simulink model "STATE_PROJECT_Harness_Test_4"  (R2022b)
settings: Solver=FixedStepAuto  StartTime=0.0  StopTime=120.0  FixedStep=0.1  RelTol=1e-3
settings Model: NumberOfSteps=10  Creator=giuse  LastModifiedBy=giuse

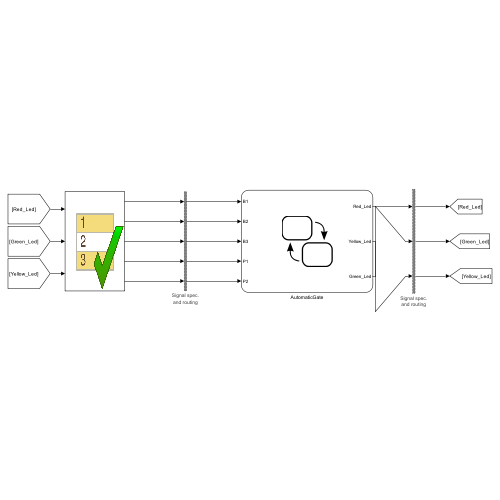
[thumbnail: Simulink's stored preview of the top-level diagram]
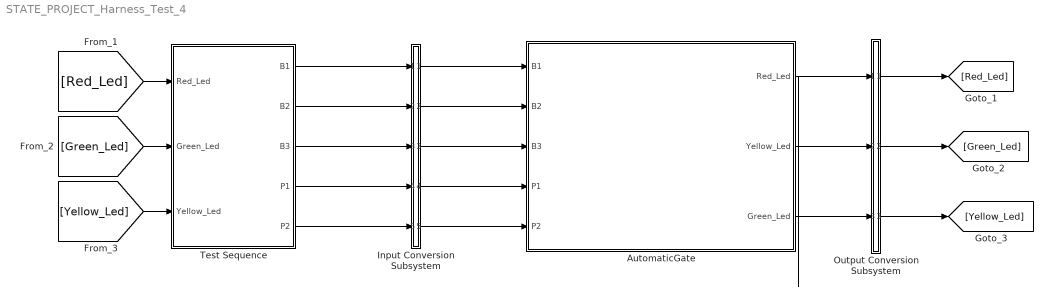
== system STATE_PROJECT_Harness_Test_4 ==
  AutomaticGate : Stateflow chart  TreatAsAtomicUnit=on
      settings: PortSchema="{\"entries\":[{\"content\":{\"sides\":[{\"content\":{\"connectorIds\":[\"In1\",\"In2\",\"In3\",\"In4\",\"In5\"]},\"type\":\"ConnectorPlacement.EquallySpacedRectSide\",\"uuid\":\"b9ac80a2-bb7a-47d7-8c7f-6386963f3ff2\"},{\"content\":{\"connectorIds\":[\"Out1\",\"Out3\",\"Out2\"],\"side\":\"RIGHT\"},\"type\":\"ConnectorPlacement.EquallySpacedRectSide\",\"uuid\":\"565990b0-d594-46a7-8ea3-0c7443a62f81\"},{\"content\":{\"connectorIds\":[],\"side\":\"TOP\"},\"type\":\"ConnectorPlacement.EquallySpacedRectSide\",\"uuid\":\"d7a99aca-bf8f-44a8-855e-79befe08fc9b\"}]},\"type\":\"ConnectorPlacement.EquallySpacedConnector\",\"uuid\":\"af0d90d0-169d-45ca-9585-d3b64258f7d0\"}],\"packageUris\":[\"http://schema.mathworks.com/mf0/Connector/R2020b\"],\"version\":\"1.0\"}"
  Input Conversion Subsystem : Subsystem  Tag=__SLT_ICS__  Description=|
      | Signal spec.
      | and routing
      settings: AttributesFormatString=%<Description>
  Output Conversion Subsystem : Subsystem  Tag=__SLT_OCS__  Description=|
      | Signal spec.
      | and routing
      settings: AttributesFormatString=%<Description>
  Test Sequence : Test Sequence  TreatAsAtomicUnit=on
  wires:
  Test Sequence/1(B1) -> Input Conversion Subsystem/1(Inport_1)
  Test Sequence/2(B2) -> Input Conversion Subsystem/2(Inport_2)
  Test Sequence/3(B3) -> Input Conversion Subsystem/3(Inport_3)
  Test Sequence/4(P1) -> Input Conversion Subsystem/4(Inport_4)
  Test Sequence/5(P2) -> Input Conversion Subsystem/5(Inport_5)
  [Red_Led] -> Test Sequence/1(Red_Led)
  [Green_Led] -> Test Sequence/2(Green_Led)
  [Yellow_Led] -> Test Sequence/3(Yellow_Led)
  Output Conversion Subsystem/1(Outport_1) -> [Red_Led]
  Output Conversion Subsystem/2(Outport_2) -> [Green_Led]
  Output Conversion Subsystem/3(Outport_3) -> [Yellow_Led]
  Input Conversion Subsystem/1(Outport_1) -> AutomaticGate/1(B1)
  Input Conversion Subsystem/2(Outport_2) -> AutomaticGate/2(B2)
  Input Conversion Subsystem/3(Outport_3) -> AutomaticGate/3(B3)
  Input Conversion Subsystem/4(Outport_4) -> AutomaticGate/4(P1)
  Input Conversion Subsystem/5(Outport_5) -> AutomaticGate/5(P2)
  AutomaticGate/1(Red_Led) -> Output Conversion Subsystem/1(Inport_1)
  AutomaticGate/2(Green_Led) -> Output Conversion Subsystem/2(Inport_2)
  AutomaticGate/3(Yellow_Led) -> Output Conversion Subsystem/3(Inport_3)

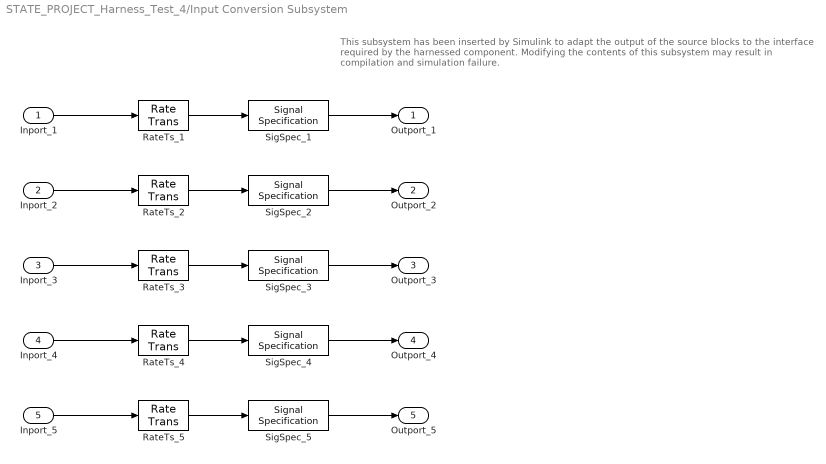
== system STATE_PROJECT_Harness_Test_4/Input Conversion Subsystem ==
  note: This subsystem has been inserted by Simulink to adapt the output of the source blocks to the interface required by the harnessed component.
      |  Modifying the contents of this subsystem may result in compilation and simulation failure.
  Inport_1 : Inport
  Inport_2 : Inport  Port=2
  Inport_3 : Inport  Port=3
  Inport_4 : Inport  Port=4
  Inport_5 : Inport  Port=5
  RateTs_{1..3,5} (4 alike) : RateTransition  OutPortSampleTime=0.1
  RateTs_4 : RateTransition  OutPortSampleTime=[-1, 0]
  SigSpec_{1..3,5} (4 alike) : SignalSpecification  OutDataTypeStr=double  Dimensions=[1]  SampleTime=0.1
  SigSpec_4 : SignalSpecification  OutDataTypeStr=double  Dimensions=[1]  SampleTime=[-1, 0]
  Outport_1 : Outport
  Outport_2 : Outport  Port=2
  Outport_3 : Outport  Port=3
  Outport_4 : Outport  Port=4
  Outport_5 : Outport  Port=5
  wires:
  SigSpec_1/1 -> Outport_1/1
  RateTs_1/1 -> SigSpec_1/1
  Inport_1/1 -> RateTs_1/1
  SigSpec_2/1 -> Outport_2/1
  RateTs_2/1 -> SigSpec_2/1
  Inport_2/1 -> RateTs_2/1
  SigSpec_3/1 -> Outport_3/1
  RateTs_3/1 -> SigSpec_3/1
  Inport_3/1 -> RateTs_3/1
  SigSpec_4/1 -> Outport_4/1
  RateTs_4/1 -> SigSpec_4/1
  Inport_4/1 -> RateTs_4/1
  SigSpec_5/1 -> Outport_5/1
  RateTs_5/1 -> SigSpec_5/1
  Inport_5/1 -> RateTs_5/1

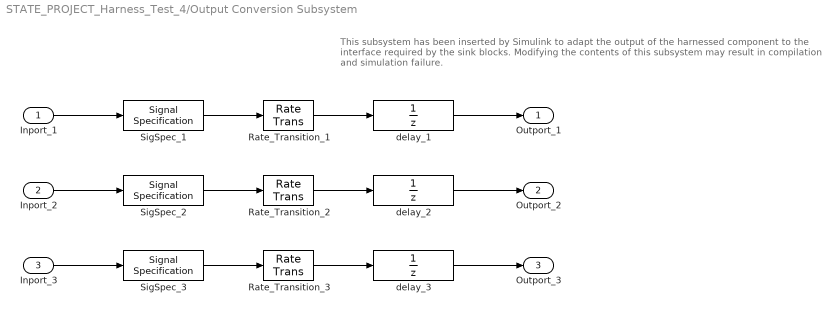
== system STATE_PROJECT_Harness_Test_4/Output Conversion Subsystem ==
  note: This subsystem has been inserted by Simulink to adapt the output of the harnessed component to the interface required by the sink blocks.
      |  Modifying the contents of this subsystem may result in compilation and simulation failure.
  Inport_1 : Inport
  Inport_2 : Inport  Port=2
  Inport_3 : Inport  Port=3
  Rate_Transition_1 : RateTransition  OutPortSampleTimeOpt=Inherit
  Rate_Transition_2 : RateTransition  OutPortSampleTimeOpt=Inherit
  Rate_Transition_3 : RateTransition  OutPortSampleTimeOpt=Inherit
  SigSpec_1 : SignalSpecification  OutDataTypeStr=double  Dimensions=[1]  SampleTime=0.1
  SigSpec_2 : SignalSpecification  OutDataTypeStr=double  Dimensions=[1]  SampleTime=0.1
  SigSpec_3 : SignalSpecification  OutDataTypeStr=double  Dimensions=[1]  SampleTime=0.1
  delay_1 : UnitDelay  SampleTime=-1
  delay_2 : UnitDelay  SampleTime=-1
  delay_3 : UnitDelay  SampleTime=-1
  Outport_1 : Outport
  Outport_2 : Outport  Port=2
  Outport_3 : Outport  Port=3
  wires:
  Inport_1/1 -> SigSpec_1/1
  SigSpec_1/1 -> Rate_Transition_1/1
  Rate_Transition_1/1 -> delay_1/1
  delay_1/1 -> Outport_1/1
  Inport_2/1 -> SigSpec_2/1
  SigSpec_2/1 -> Rate_Transition_2/1
  Rate_Transition_2/1 -> delay_2/1
  delay_2/1 -> Outport_2/1
  Inport_3/1 -> SigSpec_3/1
  SigSpec_3/1 -> Rate_Transition_3/1
  Rate_Transition_3/1 -> delay_3/1
  delay_3/1 -> Outport_3/1

== stateflow chart STATE_PROJECT_Harness_Test_4/AutomaticGate ==
  state AUTOMATIC_GATE_LOGIC
    state AUTOMATIC_GATE [parallel]
      settings: executionOrder=4
      state EMERGENCY_P1_CLOSED
        state GREEN_OFF
          en:
          Green_Led = LED_OFF;
          Yellow_Led = LED_OFF;
          Red_Led = LED_OFF;
        state GREEN_ON
          en:
          Green_Led = LED_ON;
          Yellow_Led = LED_OFF;
          Red_Led = LED_OFF;
        AUTOMATIC_GATE_LOGIC.AUTOMATIC_GATE.EMERGENCY_P1_CLOSED.GREEN_ON -> AUTOMATIC_GATE_LOGIC.AUTOMATIC_GATE.EMERGENCY_P1_CLOSED.GREEN_OFF : [after(GREEN_DUR,sec)]
        AUTOMATIC_GATE_LOGIC.AUTOMATIC_GATE.EMERGENCY_P1_CLOSED.GREEN_OFF -> AUTOMATIC_GATE_LOGIC.AUTOMATIC_GATE.EMERGENCY_P1_CLOSED.GREEN_ON : [after(GREEN_DUR,sec)]
        (default) -> AUTOMATIC_GATE_LOGIC.AUTOMATIC_GATE.EMERGENCY_P1_CLOSED.GREEN_ON
      state CLOSED
        en:
        Green_Led = LED_OFF;
        Yellow_Led = LED_OFF;
        Red_Led = LED_OFF;
        state WORK_DUR_SETTING [parallel]
          settings: executionOrder=2
          state WORK_DUR_SETTING_INTERNAL
          (default) -> WORK_DUR_SETTING_INTERNAL
          WORK_DUR_SETTING_INTERNAL -> WORK_DUR_SETTING_INTERNAL : B3_pressed{WORK_DUR = mod((WORK_DUR),120) +10;}
        state OPEN_DUR_SETTING [parallel]
          settings: executionOrder=1
          state OPEN_DUR_SETTING_INTERNAL
          OPEN_DUR_SETTING_INTERNAL -> OPEN_DUR_SETTING_INTERNAL : B2_pressed{OPEN_DUR = mod((OPEN_DUR),120) + 10;}
        (default) -> WORK_DUR_SETTING [order 2]
        (default) -> OPEN_DUR_SETTING [order 1]
      state OPENING
        state YELLOW_OFF
          en:
          Green_Led = LED_OFF;
          Yellow_Led = LED_OFF;
          Red_Led = LED_OFF;
        state YELLOW_ON
          en:
          Green_Led = LED_OFF;
          Yellow_Led = LED_ON;
          Red_Led = LED_OFF;
        AUTOMATIC_GATE_LOGIC.AUTOMATIC_GATE.OPENING.YELLOW_ON -> AUTOMATIC_GATE_LOGIC.AUTOMATIC_GATE.OPENING.YELLOW_OFF : [after(YELLOW_DUR,sec)]
        AUTOMATIC_GATE_LOGIC.AUTOMATIC_GATE.OPENING.YELLOW_OFF -> AUTOMATIC_GATE_LOGIC.AUTOMATIC_GATE.OPENING.YELLOW_ON : [after(YELLOW_DUR,sec)]
        (default) -> AUTOMATIC_GATE_LOGIC.AUTOMATIC_GATE.OPENING.YELLOW_ON
      state EMERGENCY
        en:
        Green_Led = LED_OFF;
        Yellow_Led = LED_OFF;
        Red_Led = LED_OFF;
      state EMERGENCY_LED
        en:
        Green_Led = LED_OFF;
        Yellow_Led = LED_OFF;
        Red_Led = LED_ON;
      state CLOSING
        state YELLOW_OFF
          en:
          Green_Led = LED_OFF;
          Yellow_Led = LED_OFF;
          Red_Led = LED_OFF;
        state YELLOW_ON
          en:
          Green_Led = LED_OFF;
          Yellow_Led = LED_ON;
          Red_Led = LED_OFF;
        AUTOMATIC_GATE_LOGIC.AUTOMATIC_GATE.CLOSING.YELLOW_ON -> AUTOMATIC_GATE_LOGIC.AUTOMATIC_GATE.CLOSING.YELLOW_OFF : [after(YELLOW_DUR,sec)]
        AUTOMATIC_GATE_LOGIC.AUTOMATIC_GATE.CLOSING.YELLOW_OFF -> AUTOMATIC_GATE_LOGIC.AUTOMATIC_GATE.CLOSING.YELLOW_ON : [after(YELLOW_DUR,sec)]
        (default) -> AUTOMATIC_GATE_LOGIC.AUTOMATIC_GATE.CLOSING.YELLOW_ON
      state OPEN
        en:
        Green_Led = LED_ON;
        Yellow_Led = LED_ON;
        Red_Led = LED_ON;
      state EMERGENCY_P1_OPEN
        state GREEN_OFF
          en:
          Green_Led = LED_OFF;
          Yellow_Led = LED_OFF;
          Red_Led = LED_OFF;
        state GREEN_ON
          en:
          Green_Led = LED_ON;
          Yellow_Led = LED_OFF;
          Red_Led = LED_OFF;
        AUTOMATIC_GATE_LOGIC.AUTOMATIC_GATE.EMERGENCY_P1_OPEN.GREEN_ON -> AUTOMATIC_GATE_LOGIC.AUTOMATIC_GATE.EMERGENCY_P1_OPEN.GREEN_OFF : [after(GREEN_DUR,sec)]
        AUTOMATIC_GATE_LOGIC.AUTOMATIC_GATE.EMERGENCY_P1_OPEN.GREEN_OFF -> AUTOMATIC_GATE_LOGIC.AUTOMATIC_GATE.EMERGENCY_P1_OPEN.GREEN_ON : [after(GREEN_DUR,sec)]
        (default) -> AUTOMATIC_GATE_LOGIC.AUTOMATIC_GATE.EMERGENCY_P1_OPEN.GREEN_ON
      CLOSED -> EMERGENCY_P1_CLOSED [order 1] : [B1_pressed && P1 == P_ON]
      EMERGENCY_P1_CLOSED -> CLOSED : [P1 == P_OFF || after(EMER_P1_DUR,sec)]
      CLOSED -> OPENING [order 2] : B1_pressed
      EMERGENCY -> CLOSED [order 2] : [P2 == P_ON]
      EMERGENCY_LED -> CLOSED : [P2 == P_ON]
      CLOSING -> CLOSED [order 1] : [P2 == P_ON]
      EMERGENCY -> EMERGENCY_LED [order 1] : [after(EMER_DUR,sec)]
      CLOSING -> EMERGENCY [order 3] : [after(WORK_DUR,sec)]
      OPENING -> CLOSING [order 1] : [B1_pressed && P1 == P_OFF]
      CLOSING -> OPENING [order 2] : [B1_pressed || P1 == P_ON]
      OPENING -> OPEN [order 2] : [after(WORK_DUR,sec)]
      (default) -> CLOSING
      OPEN -> CLOSING [order 1] : [after(OPEN_DUR,sec) || B1_pressed]
      EMERGENCY_P1_OPEN -> OPEN : [P1 == P_OFF || after(EMER_P1_DUR,sec)]
      OPEN -> EMERGENCY_P1_OPEN [order 2] : [B1_pressed && P1 == P_ON]
    state B1 [parallel]
      settings: executionOrder=1
      state RELEASED
      state PRESSED
      state LONGPRESSED
        send(B1_pressed)
      (default) -> AUTOMATIC_GATE_LOGIC.B1.RELEASED
      AUTOMATIC_GATE_LOGIC.B1.RELEASED -> AUTOMATIC_GATE_LOGIC.B1.PRESSED : [B1==BUTTON_ON]
      AUTOMATIC_GATE_LOGIC.B1.LONGPRESSED -> AUTOMATIC_GATE_LOGIC.B1.RELEASED : [B1 == BUTTON_OFF]
      AUTOMATIC_GATE_LOGIC.B1.PRESSED -> AUTOMATIC_GATE_LOGIC.B1.LONGPRESSED : [B1 == BUTTON_OFF]
    state B3 [parallel]
      settings: executionOrder=2
      state RELEASED
      state PRESSED
      state LONGPRESSED
        send(B3_pressed)
      (default) -> AUTOMATIC_GATE_LOGIC.B3.RELEASED
      AUTOMATIC_GATE_LOGIC.B3.RELEASED -> AUTOMATIC_GATE_LOGIC.B3.PRESSED : [B3==BUTTON_ON]
      AUTOMATIC_GATE_LOGIC.B3.LONGPRESSED -> AUTOMATIC_GATE_LOGIC.B3.RELEASED : [B3 == BUTTON_OFF]
      AUTOMATIC_GATE_LOGIC.B3.PRESSED -> AUTOMATIC_GATE_LOGIC.B3.LONGPRESSED : [B3== BUTTON_OFF]
    state B2 [parallel]
      settings: executionOrder=3
      state RELEASED
      state PRESSED
      state LONGPRESSED
        send(B2_pressed)
      (default) -> AUTOMATIC_GATE_LOGIC.B2.RELEASED
      AUTOMATIC_GATE_LOGIC.B2.RELEASED -> AUTOMATIC_GATE_LOGIC.B2.PRESSED : [B2==BUTTON_ON]
      AUTOMATIC_GATE_LOGIC.B2.LONGPRESSED -> AUTOMATIC_GATE_LOGIC.B2.RELEASED : [B2 == BUTTON_OFF]
      AUTOMATIC_GATE_LOGIC.B2.PRESSED -> AUTOMATIC_GATE_LOGIC.B2.LONGPRESSED : [B2 == BUTTON_OFF]
    (default) -> AUTOMATIC_GATE [order 1]
    (default) -> B1 [order 2]
    (default) -> B3 [order 4]
    (default) -> B2 [order 3]
  data: B1 input; B2 input; B3 input; Red_Led output; Green_Led output; Yellow_Led output; P1 input; P2 input; BUTTON_OFF constant double =0; WORK_DUR local =10; P_ON constant double =1; P_OFF constant double =0; OPEN_DUR local =10; LED_ON constant double =1; LED_OFF constant double =0; BUTTON_ON constant double =1; EMER_DUR constant double =10; YELLOW_DUR constant double =1; GREEN_DUR constant double =0.5; EMER_P1_DUR constant double =30
  events: B1_pressed local RISING_EDGE_EVENT; B2_pressed local FUNCTION_CALL_EVENT; B3_pressed local FUNCTION_CALL_EVENT

== stateflow chart STATE_PROJECT_Harness_Test_4/Test Sequence ==
  settings: updateMethod=DISCRETE  sampleTime=0.1
  state Run
    %% Initialize data outputs.
    B1 = 0;
    B2 = 0;
    B3 = 0;
    P1 = 0;
    P2 = 0;
    settings: description=Inizializzazione degli input
  state Test_closing_state
    settings: description=Test dello sato di chiusura intercendo gli stati del Led_Yellow
    state Test_closing_state_1
      verify(Yellow_Led == 1, 'TEST FAILED');
      settings: description=Yellow_Led == ON
    state Test_closing_state_2
      verify(Yellow_Led == 0, 'TEST FAILED');
      settings: description=Yellow_Led == OFF
    (default) -> Test_closing_state_1
    Test_closing_state_1 -> Test_closing_state_2 : [
        | after(1,sec)
        | ]
    Test_closing_state_2 -> Test_closing_state_1 : [
        | after(1,sec)
        | ]
  state Start_test_P1
    P1=1;
    settings: description=|
        | Inizializzazione variabile per andare nello stato di OPENING, a cusa dell'ostacolo
        | davanti a P1
  state Test_opening_state
    settings: description=Test dello sato di apertura intercendo gli stati del Led_Yellow
    state Start_test_opening_1
      verify(Yellow_Led == 1, 'TEST FAILED');
      settings: description=Yellow_Led == ON
    state Start_test_opening_2
      verify(Yellow_Led == 0, 'TEST FAILED');
      settings: description=Yellow_Led == OFF
    (default) -> Start_test_opening_1
    Start_test_opening_1 -> Start_test_opening_2 : [
        | after(1,sec)
        | ]
    Start_test_opening_2 -> Start_test_opening_1 : [
        | after(1,sec)
        | ]
  state Test_open_state
    verify(Green_Led == 1, 'TEST FAILED');
    verify(Yellow_Led == 1, 'TEST FAILED');
    verify(Red_Led == 1, 'TEST FAILED');
    settings: description=Testinf dello stato OPEN verificando che tutti i led sono accesi
  state Test_change_P1
    P1=0;
    settings: description=Inizializzazione sensore P1 a 0 per togliere l'ostacolo
  state Start_test_closing_state
    settings: description="Genera fronte di salita e discesa del pulsante B1 per cambiare da stato OPEN  A CLOSING"
    state Start_test_closing_state_1
      B1=1;
      settings: description=B1 = 1
    state Start_test_closing_state_2
      B1=0;
      settings: description=B1 = 0
    (default) -> Start_test_closing_state_1
    Start_test_closing_state_1 -> Start_test_closing_state_2 : [
        | after(0.1,sec)
        | ]
    Start_test_closing_state_2 -> Start_test_closing_state_1 : [
        | after(0.1,sec)
        | ]
  (default) -> Run
  Run -> Test_closing_state
  (junction 97) -> Test_closing_state
  (junction 99) -> (junction 97)
  Test_closing_state -> Start_test_P1 : [
      | after(5,sec)
      | ]
  Start_test_P1 -> Test_opening_state : [
      | true
      | ]
  Test_opening_state -> Test_open_state : [
      | after(10,sec)
      | ]
  Test_open_state -> Test_change_P1 : [
      | after(1,sec)
      | ]
  Test_change_P1 -> Start_test_closing_state : [
      | true
      | ]
  Start_test_closing_state -> (junction 99) : [
      | after(0.2,sec)
      | ]
  data: Red_Led input double size=[1]; Green_Led input double size=[1]; Yellow_Led input double size=[1]; B1 output double size=[1]; B2 output double size=[1]; B3 output double size=[1]; P1 output double size=[1]; P2 output double size=[1]
